simulink library "IOBlock_Library_TTC580"  (R2021a)
settings: Solver=ode45  StartTime=0.0  StopTime=10.0  RelTol=1e-3
PreLoadFcn:
  | addpath(genpath(fileparts(which('IOBlock_Library_TTC580'))));
  | %addpath(genpath(fileparts(which('IOBlock_Library_TTC580.mdl'))))
  | try
  | addpath(genpath([fileparts(which('IOBlock_Library_TTC580')),'\..\DBC_Importer']));
  | addpath(genpath([fileparts(which('IOBlock_Library_TTC580')),'\..\EEPROM_Importer']));
  | addpath(genpath([fileparts(which('IOBlock_Library_TTC580')),'\..\UserDoc']));
  | catch
  | warning('IOBlock_Library_TTC580: add path to DBC_Importer and EEPROM_Importer manually');
  | end
  | try
  | if exist('..\CustomPackage\scripts\OpenAllPackages.m','file')
  |      run('..\CustomPackage\scripts\OpenAllPackages.m'); %always available, ggf. empty
  | end
  | catch
  | warning('A problem occurred opening automatically the CustomPackage. Please open libraries manually');
  | end
  | try
  | set_param(0,'EditorSmartEditingHotParam','off');
  | catch
  | warning('Simlink preferences for ''Edit key parameter when adding new blocks'' needs to be unchecked manually');
  | end
undefined symbols (not defined in the file or in its folder): ADC_Absolute_10V, ADC_Absolute_32V, ADC_Absolute_5V, ADC_BoardTemp, ADC_ChannelInit, ADC_Current, ADC_Get, ADC_K15_, ADC_Ratiometric_10V, ADC_Ratiometric_5V, ADC_Resistive, ADC_SensorSupply, ADC_UBAT, bit_packing, bit_unpacking, CAN_ConfigMsg, compare2error, compare2FET_PROT_REENABLE, crc32_calc_intern, CRC32_EEPROM_Read, CRC32_EEPROM_Write, DIAG_EnterSafestate, DIAG_Status, DIAG_Status_internal, EEPROM_Mirror, EEPROM_Read, EEPROM_Read_OffsetIn, EEPROM_Read_Raw, EEPROM_Write, EEPROM_Write_OffsetIn, EEPROM_Write_Raw, EnterSafestate, FPU_Handler, Get_DI, Get_DI_VarThreshold, Get_K15_, Get_Pulse_Freq_Curr, Get_Pulse_Freq_Volt, Get_WakeUp, GetDateAndTime, IO_ADC_ResetProtection, IO_Blk_Lib_TTC500, IO_CAN_ReadMsg, IO_CAN_WriteMsg, IO_DI_Get, IO_DI_Init, IO_DI_Init_Var, IO_DO_GetCur, IO_DO_GetVoltage, IO_DO_Init, IO_DO_ResetProtection, IO_DO_Set, IO_Driver_GetSerialNumber, IO_Driver_GetVersionOfDriver, IO_Driver_GetVersionOfFPGA, IO_EEPROM_GetStatus, IO_EEPROM_Init, IO_EEPROM_Read_raw, IO_EEPROM_Write, IO_EEPROM_Write_OffsetIn ... (+73)
libraries: simulink x43
(part 10 of 18)

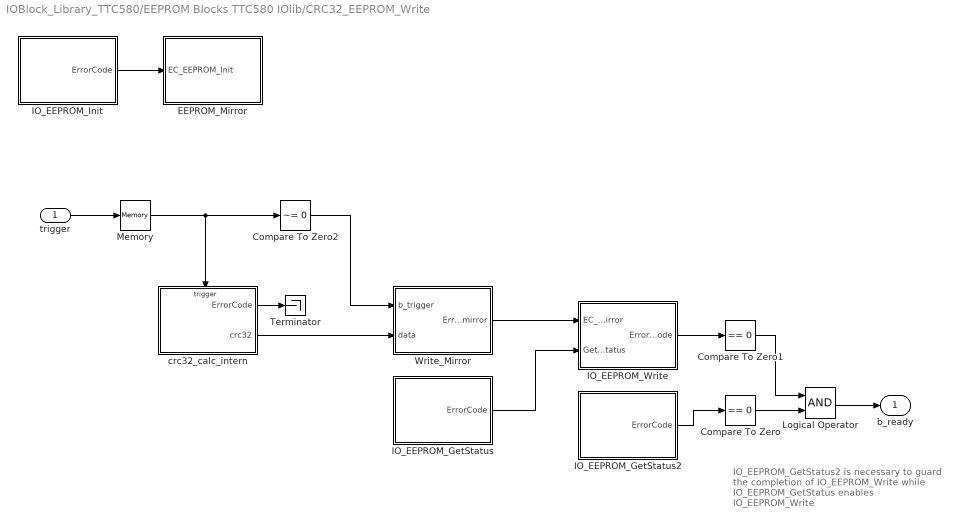
== system IOBlock_Library_TTC580/EEPROM Blocks TTC580 IOlib/CRC32_EEPROM_Write ==
  note: IO_EEPROM_GetStatus2 is necessary to
      | guard the completion of IO_EEPROM_Write
      | while IO_EEPROM_GetStatus enables
      | IO_EEPROM_Write
  trigger : Inport
  Compare To Zero : simulink/Logic and Bit Operations/Compare To Zero  relop===  OutDataTypeStr=boolean  ZeroCross=off
  Compare To Zero1 : simulink/Logic and Bit Operations/Compare To Zero  relop===  OutDataTypeStr=boolean  ZeroCross=off
  Compare To Zero2 : simulink/Logic and Bit Operations/Compare To Zero  relop=~=  OutDataTypeStr=boolean  ZeroCross=off
  EEPROM_Mirror : Subsystem  LoadFcn=|  mask(EEPROM_Mirror_Code){SampleTime=-1, ttlib=IO_Blk_Lib_TTC500, ttDescription=EEPROM_Mirror, tt_iolib_version=0.21, offset=0, length=65536}
      | try
      | %
      | %Upgrade Information - standard BEGIN
      | new_color = 'blue';
      | new_ver = '0.21';
      | act_ver = get_param(gcb,'tt_iolib_version');
      | if not(strcmp(act_ver,new_ver))
      |     disp(['Upgrade block: ',gcb,char(10),'       Version: ',act_ver,' -> ',new_ver]);
      |     %switch - case for specific upgrade information e.g. additional parameter required 
      |     %Change appearance and version information
      |     set_param(gcb,'ForegroundColor',new_color);
      |     set_param(gcb,'tt_iolib_version',new_ver);
      | end
      | %Upgrade Information - standard END
      | catch
      | %Standard catch section BEGIN 
      | disp(' ');
      | disp('------------------------------------------------------------');
      | disp('An error occurred in a callback of the TTC580-BlockLib.');
      | disp(['Please check the parameters in the mask of ',gcb]);
      | disp('If you do not encounter any violations, then please '); 
      | disp('copy the following lines and report this to support@ttcontrol.com ');
      | disp('<< begin of error message dump >>');
      | disp(['Version of TTC580-BlockLib: ', get_param(gcb,'tt_iolib_version')]);
      | disp(get_param(gcb,'ttDescription'));
      | disp(gcb);
      | x=lasterror;disp(x.message);
      | disp(get_param(gcb,'MaskValues'));
      | disp(version);
      | disp(computer);
      | disp('<< end of error message dump >>');
      | disp('------------------------------------------------------------');
      | disp(' ');
      | %Standard catch section END
      | end
      mask help:
      | Read all data from the EEPROM and mirror this onto RAM.
      | The ErrorCode of IO_EEPROM_Init - block must be connected to the input of EEPROM_Mirror.
      | After calling EEPROM_Mirror the global variable EEPROM_mirror is filled and
      | the global variable ErrorCode_EEPROM_mirror contains the returns of IO_EEPROM_Init() and IO_EEPROM_Read().
      mask init:
      | %
      settings: CopyFcn=%deleted
      mask Help: web(which('IO_EEPROM.h'))
      mask Callback offset: %
      mask Callback length: %
  IO_EEPROM_GetStatus : Subsystem  LoadFcn=|  mask(IO_EEPROM_GetStatus_Code){SampleTime=-1, ttlib=IO_Blk_Lib_TTC500, ttDescription=IO_EEPROM_GetStatus, tt_iolib_version=0.19}
      | try
      | %
      | %Upgrade Information - standard BEGIN
      | new_color = 'blue';
      | new_ver = '0.19';
      | act_ver = get_param(gcb,'tt_iolib_version');
      | if not(strcmp(act_ver,new_ver))
      |     disp(['Upgrade block: ',gcb,char(10),'       Version: ',act_ver,' -> ',new_ver]);
      |     %switch - case for specific upgrade information e.g. additional parameter required 
      |     %Change appearance and version information
      |     set_param(gcb,'ForegroundColor',new_color);
      |     set_param(gcb,'tt_iolib_version',new_ver);
      | end
      | %Upgrade Information - standard END
      | catch
      | %Standard catch section BEGIN 
      | disp(' ');
      | disp('------------------------------------------------------------');
      | disp('An error occurred in a callback of the TTC580-BlockLib.');
      | disp(['Please check the parameters in the mask of ',gcb]);
      | disp('If you do not encounter any violations, then please '); 
      | disp('copy the following lines and report this to support@ttcontrol.com ');
      | disp('<< begin of error message dump >>');
      | disp(['Version of TTC580-BlockLib: ', get_param(gcb,'tt_iolib_version')]);
      | disp(get_param(gcb,'ttDescription'));
      | disp(gcb);
      | x=lasterror;disp(x.message);
      | disp(get_param(gcb,'MaskValues'));
      | disp(version);
      | disp(computer);
      | disp('<< end of error message dump >>');
      | disp('------------------------------------------------------------');
      | disp(' ');
      | %Standard catch section END
      | end
      mask help: Returns the status of the EEPROM driver.
      mask init:
      | %
      settings: CopyFcn=%deleted
      mask Help: web(which('IO_EEPROM.h'))
  IO_EEPROM_GetStatus2 : Subsystem  LoadFcn=|  mask(IO_EEPROM_GetStatus_Code){SampleTime=-1, ttlib=IO_Blk_Lib_TTC500, ttDescription=IO_EEPROM_GetStatus, tt_iolib_version=0.19}
      | try
      | %
      | %Upgrade Information - standard BEGIN
      | new_color = 'blue';
      | new_ver = '0.19';
      | act_ver = get_param(gcb,'tt_iolib_version');
      | if not(strcmp(act_ver,new_ver))
      |     disp(['Upgrade block: ',gcb,char(10),'       Version: ',act_ver,' -> ',new_ver]);
      |     %switch - case for specific upgrade information e.g. additional parameter required 
      |     %Change appearance and version information
      |     set_param(gcb,'ForegroundColor',new_color);
      |     set_param(gcb,'tt_iolib_version',new_ver);
      | end
      | %Upgrade Information - standard END
      | catch
      | %Standard catch section BEGIN 
      | disp(' ');
      | disp('------------------------------------------------------------');
      | disp('An error occurred in a callback of the TTC580-BlockLib.');
      | disp('Please copy the following lines and report this to support@tttech.com ');
      | disp('<< begin of error message dump >>');
      | disp(['Version of TTC580-BlockLib: ', get_param(gcb,'tt_iolib_version')]);
      | disp(get_param(gcb,'ttDescription'));
      | disp(gcb);
      | x=lasterror;disp(x.message);
      | disp(get_param(gcb,'MaskValues'));
      | disp(version);
      | disp(computer);
      | disp('<< end of error message dump >>');
      | disp('------------------------------------------------------------');
      | disp(' ');
      | %Standard catch section END
      | end
      mask help: Returns the status of the EEPROM driver.
      mask init:
      | %
      settings: CopyFcn=%deleted
      mask Help: web(which('IO_EEPROM.h'))
  IO_EEPROM_Init : Subsystem  LoadFcn=|  mask(IO_EEPROM_Init_Code){SampleTime=-1, ttlib=IO_Blk_Lib_TTC500, ttDescription=IO_EEPROM_Init, tt_iolib_version=0.19}
      | try
      | %
      | %Upgrade Information - standard BEGIN
      | new_color = 'blue';
      | new_ver = '0.19';
      | act_ver = get_param(gcb,'tt_iolib_version');
      | if not(strcmp(act_ver,new_ver))
      |     disp(['Upgrade block: ',gcb,char(10),'       Version: ',act_ver,' -> ',new_ver]);
      |     %switch - case for specific upgrade information e.g. additional parameter required 
      |     %Change appearance and version information
      |     set_param(gcb,'ForegroundColor',new_color);
      |     set_param(gcb,'tt_iolib_version',new_ver);
      | end
      | %Upgrade Information - standard END
      | catch
      | %Standard catch section BEGIN 
      | disp(' ');
      | disp('------------------------------------------------------------');
      | disp('An error occurred in a callback of the TTC580-BlockLib.');
      | disp(['Please check the parameters in the mask of ',gcb]);
      | disp('If you do not encounter any violations, then please '); 
      | disp('copy the following lines and report this to support@ttcontrol.com ');
      | disp('<< begin of error message dump >>');
      | disp(['Version of TTC580-BlockLib: ', get_param(gcb,'tt_iolib_version')]);
      | disp(get_param(gcb,'ttDescription'));
      | disp(gcb);
      | x=lasterror;disp(x.message);
      | disp(get_param(gcb,'MaskValues'));
      | disp(version);
      | disp(computer);
      | disp('<< end of error message dump >>');
      | disp('------------------------------------------------------------');
      | disp(' ');
      | %Standard catch section END
      | end
      mask help: Initialization of the EEPROM driver.
      mask init:
      | %
      settings: CopyFcn=%deleted
      mask Help: web(which('IO_EEPROM.h'))
  IO_EEPROM_Write : Subsystem  LoadFcn=|  mask(IO_EEPROM_Write_Code){SampleTime=-1, ttlib=IO_Blk_Lib_TTC500, ttDescription=IO_EEPROM_Write, tt_iolib_version=0.19, offset=offset, length=length}
      | try
      | %
      | %Upgrade Information - standard BEGIN
      | new_color = 'blue';
      | new_ver = '0.19';
      | act_ver = get_param(gcb,'tt_iolib_version');
      | if not(strcmp(act_ver,new_ver))
      |     disp(['Upgrade block: ',gcb,char(10),'       Version: ',act_ver,' -> ',new_ver]);
      |     %switch - case for specific upgrade information e.g. additional parameter required 
      |     %Change appearance and version information
      |     set_param(gcb,'ForegroundColor',new_color);
      |     set_param(gcb,'tt_iolib_version',new_ver);
      | end
      | %Upgrade Information - standard END
      | catch
      | %Standard catch section BEGIN 
      | disp(' ');
      | disp('------------------------------------------------------------');
      | disp('An error occurred in a callback of the TTC580-BlockLib.');
      | disp(['Please check the parameters in the mask of ',gcb]);
      | disp('If you do not encounter any violations, then please '); 
      | disp('copy the following lines and report this to support@ttcontrol.com ');
      | disp('<< begin of error message dump >>');
      | disp(['Version of TTC580-BlockLib: ', get_param(gcb,'tt_iolib_version')]);
      | disp(get_param(gcb,'ttDescription'));
      | disp(gcb);
      | x=lasterror;disp(x.message);
      | disp(get_param(gcb,'MaskValues'));
      | disp(version);
      | disp(computer);
      | disp('<< end of error message dump >>');
      | disp('------------------------------------------------------------');
      | disp(' ');
      | %Standard catch section END
      | end
      mask help:
      | Copy data from EEPROM_mirror[] to physical EEPROM. Copy activity is triggered by the edge of the input "EC_Write_Mirror" from IO_E_BUSY to IO_E_OK.
      | The output "ErrorCode" is IO_E_BUSY as long as writing to EEPROM is pending. During the activities are performed writing to the physical EEPROM, "ErrorCode" corresponds to the output of the C-driver IO_EEPROM_Write().
      mask init:
      | %
      settings: CopyFcn=%deleted
      mask Help: web(which('IO_EEPROM.h'))
      mask Callback offset: %
      mask Callback length: %
  Logical Operator : Logic  AllPortsSameDT=off  OutDataTypeStr=boolean
  Memory : Memory  LinearizeAsDelay=on
  Terminator : Terminator
  Write_Mirror : Subsystem  LoadFcn=|  mask(Write_Mirror_Code){SampleTime=-1, ttlib=IO_Blk_Lib_TTC500, ttDescription=Write_Mirror, tt_iolib_version=0.19, offset=offset, length=length}
      | try
      | %
      | %Upgrade Information - standard BEGIN
      | new_color = 'blue';
      | new_ver = '0.19';
      | act_ver = get_param(gcb,'tt_iolib_version');
      | if not(strcmp(act_ver,new_ver))
      |     disp(['Upgrade block: ',gcb,char(10),'       Version: ',act_ver,' -> ',new_ver]);
      |     %switch - case for specific upgrade information e.g. additional parameter required 
      |     %Change appearance and version information
      |     set_param(gcb,'ForegroundColor',new_color);
      |     set_param(gcb,'tt_iolib_version',new_ver);
      | end
      | %Upgrade Information - standard END
      | catch
      | %Standard catch section BEGIN 
      | disp(' ');
      | disp('------------------------------------------------------------');
      | disp('An error occurred in a callback of the TTC580-BlockLib.');
      | disp(['Please check the parameters in the mask of ',gcb]);
      | disp('If you do not encounter any violations, then please '); 
      | disp('copy the following lines and report this to support@ttcontrol.com ');
      | disp('<< begin of error message dump >>');
      | disp(['Version of TTC580-BlockLib: ', get_param(gcb,'tt_iolib_version')]);
      | disp(get_param(gcb,'ttDescription'));
      | disp(gcb);
      | x=lasterror;disp(x.message);
      | disp(get_param(gcb,'MaskValues'));
      | disp(version);
      | disp(computer);
      | disp('<< end of error message dump >>');
      | disp('------------------------------------------------------------');
      | disp(' ');
      | %Standard catch section END
      | end
      mask help:
      | Write data to the mirror of the EEPROM. ErrorCode is set to IO_E_BUSY for one cycle of writing into EEPROM_mirror[].
      | In case the given data section exceeds given EEPROM boundaries, IO_E_EEPROM_RANGE ErrorCode is returned.
      mask init:
      | %
      settings: CopyFcn=%deleted
      mask Help: web(which('~.h'))
      mask Callback offset: %
      mask Callback length: %
  crc32_calc_intern : Subsystem  LoadFcn=|  mask(crc32_calc_intern_Code){SampleTime=-1, ttlib=IO_Blk_Lib_TTC500, ttDescription=crc32_calc_intern, tt_iolib_version=0.19, EEPROM_mirror=EEPROM_mirror, iBasicAddr_intern=BasicAddr, iEndAddr_intern=EndAddr}
      | try
      | %
      | %Upgrade Information - standard BEGIN
      | new_color = 'blue';
      | new_ver = '0.19';
      | act_ver = get_param(gcb,'tt_iolib_version');
      | if not(strcmp(act_ver,new_ver))
      |     disp(['Upgrade block: ',gcb,char(10),'       Version: ',act_ver,' -> ',new_ver]);
      |     %switch - case for specific upgrade information e.g. additional parameter required 
      |     %Change appearance and version information
      |     set_param(gcb,'ForegroundColor',new_color);
      |     set_param(gcb,'tt_iolib_version',new_ver);
      | end
      | %Upgrade Information - standard END
      | catch
      | %Standard catch section BEGIN 
      | disp(' ');
      | disp('------------------------------------------------------------');
      | disp('An error occurred in a callback of the TTC580-BlockLib.');
      | disp(['Please check the parameters in the mask of ',gcb]);
      | disp('If you do not encounter any violations, then please '); 
      | disp('copy the following lines and report this to support@ttcontrol.com ');
      | disp('<< begin of error message dump >>');
      | disp(['Version of TTC580-BlockLib: ', get_param(gcb,'tt_iolib_version')]);
      | disp(get_param(gcb,'ttDescription'));
      | disp(gcb);
      | x=lasterror;disp(x.message);
      | disp(get_param(gcb,'MaskValues'));
      | disp(version);
      | disp(computer);
      | disp('<< end of error message dump >>');
      | disp('------------------------------------------------------------');
      | disp(' ');
      | %Standard catch section END
      | end
      mask help:
      | Calculate crc32 for a section out of the EEPROM.
      | In case the given data section exceeds given EEPROM boundaries, non zero ErrorCode is returned.
      mask init:
      | %
      settings: CopyFcn=%deleted
      mask Help: No further help available for this block
      mask Callback EEPROM_mirror: %
      mask Callback iBasicAddr_intern: %
      mask Callback iEndAddr_intern: %
  b_ready : Outport  VectorParamsAs1DForOutWhenUnconnected=off
  wires:
  IO_EEPROM_GetStatus2/1(ErrorCode) -> Compare To Zero/1
  Compare To Zero/1 -> Logical Operator/2
  crc32_calc_intern/1(ErrorCode) -> Terminator/1
  Logical Operator/1 -> b_ready/1
  Compare To Zero1/1 -> Logical Operator/1
  Memory/1 -> crc32_calc_intern/Trigger, Compare To Zero2/1
  Compare To Zero2/1 -> Write_Mirror/1(b_trigger)
  crc32_calc_intern/2(crc32) -> Write_Mirror/2(data)
  IO_EEPROM_GetStatus/1(ErrorCode) -> IO_EEPROM_Write/2(GetStatus)
  Write_Mirror/1(ErrorCode_EEPROM_mirror) -> IO_EEPROM_Write/1(EC_Write_Mirror)
  trigger/1 -> Memory/1
  IO_EEPROM_Write/1(ErrorCode) -> Compare To Zero1/1
  IO_EEPROM_Init/1(ErrorCode) -> EEPROM_Mirror/1(EC_EEPROM_Init)

== system IOBlock_Library_TTC580/EEPROM Blocks TTC580 IOlib/EEPROM_Read ==
  Compare To Zero1 : simulink/Logic and Bit Operations/Compare To Zero  relop===  OutDataTypeStr=boolean  ZeroCross=off
  Compare To Zero2 : simulink/Logic and Bit Operations/Compare To Zero  relop===  OutDataTypeStr=boolean  ZeroCross=off
  EEPROM_Mirror : Subsystem  LoadFcn=|  mask(EEPROM_Mirror_Code){SampleTime=-1, ttlib=IO_Blk_Lib_TTC500, ttDescription=EEPROM_Mirror, tt_iolib_version=0.21, offset=0, length=65536}
      | try
      | %
      | %Upgrade Information - standard BEGIN
      | new_color = 'blue';
      | new_ver = '0.21';
      | act_ver = get_param(gcb,'tt_iolib_version');
      | if not(strcmp(act_ver,new_ver))
      |     disp(['Upgrade block: ',gcb,char(10),'       Version: ',act_ver,' -> ',new_ver]);
      |     %switch - case for specific upgrade information e.g. additional parameter required 
      |     %Change appearance and version information
      |     set_param(gcb,'ForegroundColor',new_color);
      |     set_param(gcb,'tt_iolib_version',new_ver);
      | end
      | %Upgrade Information - standard END
      | catch
      | %Standard catch section BEGIN 
      | disp(' ');
      | disp('------------------------------------------------------------');
      | disp('An error occurred in a callback of the TTC580-BlockLib.');
      | disp(['Please check the parameters in the mask of ',gcb]);
      | disp('If you do not encounter any violations, then please '); 
      | disp('copy the following lines and report this to support@ttcontrol.com ');
      | disp('<< begin of error message dump >>');
      | disp(['Version of TTC580-BlockLib: ', get_param(gcb,'tt_iolib_version')]);
      | disp(get_param(gcb,'ttDescription'));
      | disp(gcb);
      | x=lasterror;disp(x.message);
      | disp(get_param(gcb,'MaskValues'));
      | disp(version);
      | disp(computer);
      | disp('<< end of error message dump >>');
      | disp('------------------------------------------------------------');
      | disp(' ');
      | %Standard catch section END
      | end
      mask help:
      | Read all data from the EEPROM and mirror this onto RAM.
      | The ErrorCode of IO_EEPROM_Init - block must be connected to the input of EEPROM_Mirror.
      | After calling EEPROM_Mirror the global variable EEPROM_mirror is filled and
      | the global variable ErrorCode_EEPROM_mirror contains the returns of IO_EEPROM_Init() and IO_EEPROM_Read().
      mask init:
      | %
      settings: CopyFcn=%deleted
      mask Help: web(which('IO_EEPROM.h'))
      mask Callback offset: %
      mask Callback length: %
  IO_EEPROM_GetStatus : Subsystem  LoadFcn=|  mask(IO_EEPROM_GetStatus_Code){SampleTime=-1, ttlib=IO_Blk_Lib_TTC500, ttDescription=IO_EEPROM_GetStatus, tt_iolib_version=0.19}
      | try
      | %
      | %Upgrade Information - standard BEGIN
      | new_color = 'blue';
      | new_ver = '0.19';
      | act_ver = get_param(gcb,'tt_iolib_version');
      | if not(strcmp(act_ver,new_ver))
      |     disp(['Upgrade block: ',gcb,char(10),'       Version: ',act_ver,' -> ',new_ver]);
      |     %switch - case for specific upgrade information e.g. additional parameter required 
      |     %Change appearance and version information
      |     set_param(gcb,'ForegroundColor',new_color);
      |     set_param(gcb,'tt_iolib_version',new_ver);
      | end
      | %Upgrade Information - standard END
      | catch
      | %Standard catch section BEGIN 
      | disp(' ');
      | disp('------------------------------------------------------------');
      | disp('An error occurred in a callback of the TTC580-BlockLib.');
      | disp(['Please check the parameters in the mask of ',gcb]);
      | disp('If you do not encounter any violations, then please '); 
      | disp('copy the following lines and report this to support@ttcontrol.com ');
      | disp('<< begin of error message dump >>');
      | disp(['Version of TTC580-BlockLib: ', get_param(gcb,'tt_iolib_version')]);
      | disp(get_param(gcb,'ttDescription'));
      | disp(gcb);
      | x=lasterror;disp(x.message);
      | disp(get_param(gcb,'MaskValues'));
      | disp(version);
      | disp(computer);
      | disp('<< end of error message dump >>');
      | disp('------------------------------------------------------------');
      | disp(' ');
      | %Standard catch section END
      | end
      mask help: Returns the status of the EEPROM driver.
      mask init:
      | %
      settings: CopyFcn=%deleted
      mask Help: web(which('IO_EEPROM.h'))
  IO_EEPROM_Init : Subsystem  LoadFcn=|  mask(IO_EEPROM_Init_Code){SampleTime=-1, ttlib=IO_Blk_Lib_TTC500, ttDescription=IO_EEPROM_Init, tt_iolib_version=0.19}
      | try
      | %
      | %Upgrade Information - standard BEGIN
      | new_color = 'blue';
      | new_ver = '0.19';
      | act_ver = get_param(gcb,'tt_iolib_version');
      | if not(strcmp(act_ver,new_ver))
      |     disp(['Upgrade block: ',gcb,char(10),'       Version: ',act_ver,' -> ',new_ver]);
      |     %switch - case for specific upgrade information e.g. additional parameter required 
      |     %Change appearance and version information
      |     set_param(gcb,'ForegroundColor',new_color);
      |     set_param(gcb,'tt_iolib_version',new_ver);
      | end
      | %Upgrade Information - standard END
      | catch
      | %Standard catch section BEGIN 
      | disp(' ');
      | disp('------------------------------------------------------------');
      | disp('An error occurred in a callback of the TTC580-BlockLib.');
      | disp(['Please check the parameters in the mask of ',gcb]);
      | disp('If you do not encounter any violations, then please '); 
      | disp('copy the following lines and report this to support@ttcontrol.com ');
      | disp('<< begin of error message dump >>');
      | disp(['Version of TTC580-BlockLib: ', get_param(gcb,'tt_iolib_version')]);
      | disp(get_param(gcb,'ttDescription'));
      | disp(gcb);
      | x=lasterror;disp(x.message);
      | disp(get_param(gcb,'MaskValues'));
      | disp(version);
      | disp(computer);
      | disp('<< end of error message dump >>');
      | disp('------------------------------------------------------------');
      | disp(' ');
      | %Standard catch section END
      | end
      mask help: Initialization of the EEPROM driver.
      mask init:
      | %
      settings: CopyFcn=%deleted
      mask Help: web(which('IO_EEPROM.h'))
  Logical Operator : Logic  AllPortsSameDT=off  OutDataTypeStr=boolean
  Read_Mirror : Subsystem  LoadFcn=|  mask(Read_Mirror_Code){SampleTime=-1, ttlib=IO_Blk_Lib_TTC500, ttDescription=Read_Mirror, tt_iolib_version=0.19, offset=offset, length=length}
      | try
      | %
      | %Upgrade Information - standard BEGIN
      | new_color = 'blue';
      | new_ver = '0.19';
      | act_ver = get_param(gcb,'tt_iolib_version');
      | if not(strcmp(act_ver,new_ver))
      |     disp(['Upgrade block: ',gcb,char(10),'       Version: ',act_ver,' -> ',new_ver]);
      |     %switch - case for specific upgrade information e.g. additional parameter required 
      |     %Change appearance and version information
      |     set_param(gcb,'ForegroundColor',new_color);
      |     set_param(gcb,'tt_iolib_version',new_ver);
      | end
      | %Upgrade Information - standard END
      | catch
      | %Standard catch section BEGIN 
      | disp(' ');
      | disp('------------------------------------------------------------');
      | disp('An error occurred in a callback of the TTC580-BlockLib.');
      | disp(['Please check the parameters in the mask of ',gcb]);
      | disp('If you do not encounter any violations, then please '); 
      | disp('copy the following lines and report this to support@ttcontrol.com ');
      | disp('<< begin of error message dump >>');
      | disp(['Version of TTC580-BlockLib: ', get_param(gcb,'tt_iolib_version')]);
      | disp(get_param(gcb,'ttDescription'));
      | disp(gcb);
      | x=lasterror;disp(x.message);
      | disp(get_param(gcb,'MaskValues'));
      | disp(version);
      | disp(computer);
      | disp('<< end of error message dump >>');
      | disp('------------------------------------------------------------');
      | disp(' ');
      | %Standard catch section END
      | end
      mask help:
      | Read data from the mirror of the EEPROM.
      | In case the given data section exceeds given EEPROM boundaries, IO_E_EEPROM_RANGE ErrorCode is returned.
      mask init:
      | %
      settings: CopyFcn=%deleted
      mask Help: web(which('~.h'))
      mask Callback offset: %
      mask Callback length: %
  once_true: Mirror filled : Subsystem  mask(SRFlipFlop){initial_condition=0}
      mask prompts: initial_condition "Initial condition (state of Q):"
      mask help: S-R Flip-Flop Block
      mask Help:
      | The S-R flip-flop also known as a set-reset flip-flop. This implementation
      | is modeled after an S-R flip-flop constructed using NOR gates. The
      | truth table for this block is:
      | <pre>
      |  S  R   Q  !Q
      |  ----------------
      |  1  0   1  0
      |  0  0   1  0  (after S == 1, R == 0)
      |  0  1   0  1
      |  0  0   0  1  (after S == 0, R == 1)
      |  1  1   0  0
      | </pre>
      | 
      | In an S-R flip-flop that is implemented with NOR gates, when a 1 is
      | applied to both the set and reset inputs, both outputs go to 0. Technically,
      | this state is undefined and is usually avoided. Note, if the flip-flop is
      | implemented with NAND gates, when a 0 is applied to both inputs, both outputs
      | go to 0 and when a 1 is applied to both inputs, the output depends on
      | the previous state of the flip-flop (previous value of Q).
  b_ready : Outport  VectorParamsAs1DForOutWhenUnconnected=off
  data : Outport  Port=2  OutDataTypeStr=EEPROM_type  VectorParamsAs1DForOutWhenUnconnected=off
  wires:
  Read_Mirror/2(data) -> data/1
  Read_Mirror/1(ErrorCode_EEPROM_mirror) -> Compare To Zero1/1
  IO_EEPROM_Init/1(ErrorCode) -> EEPROM_Mirror/1(EC_EEPROM_Init)
  IO_EEPROM_GetStatus/1(ErrorCode) -> Compare To Zero2/1
  Logical Operator/1 -> b_ready/1
  Compare To Zero1/1 -> Logical Operator/2
  Compare To Zero2/1 -> once_true: Mirror filled/1(S)
  once_true: Mirror filled/1(Q) -> Logical Operator/1

== system IOBlock_Library_TTC580/EEPROM Blocks TTC580 IOlib/EEPROM_Read_OffsetIn ==
  offset : Inport  OutDataTypeStr=uint16  PortDimensions=1
  Compare To Zero1 : simulink/Logic and Bit Operations/Compare To Zero  relop===  OutDataTypeStr=boolean  ZeroCross=off
  Compare To Zero2 : simulink/Logic and Bit Operations/Compare To Zero  relop===  OutDataTypeStr=boolean  ZeroCross=off
  EEPROM_Mirror : Subsystem  LoadFcn=|  mask(EEPROM_Mirror_Code){SampleTime=-1, ttlib=IO_Blk_Lib_TTC500, ttDescription=EEPROM_Mirror, tt_iolib_version=0.21, offset=0, length=65536}
      | try
      | %
      | %Upgrade Information - standard BEGIN
      | new_color = 'blue';
      | new_ver = '0.21';
      | act_ver = get_param(gcb,'tt_iolib_version');
      | if not(strcmp(act_ver,new_ver))
      |     disp(['Upgrade block: ',gcb,char(10),'       Version: ',act_ver,' -> ',new_ver]);
      |     %switch - case for specific upgrade information e.g. additional parameter required 
      |     %Change appearance and version information
      |     set_param(gcb,'ForegroundColor',new_color);
      |     set_param(gcb,'tt_iolib_version',new_ver);
      | end
      | %Upgrade Information - standard END
      | catch
      | %Standard catch section BEGIN 
      | disp(' ');
      | disp('------------------------------------------------------------');
      | disp('An error occurred in a callback of the TTC580-BlockLib.');
      | disp(['Please check the parameters in the mask of ',gcb]);
      | disp('If you do not encounter any violations, then please '); 
      | disp('copy the following lines and report this to support@ttcontrol.com ');
      | disp('<< begin of error message dump >>');
      | disp(['Version of TTC580-BlockLib: ', get_param(gcb,'tt_iolib_version')]);
      | disp(get_param(gcb,'ttDescription'));
      | disp(gcb);
      | x=lasterror;disp(x.message);
      | disp(get_param(gcb,'MaskValues'));
      | disp(version);
      | disp(computer);
      | disp('<< end of error message dump >>');
      | disp('------------------------------------------------------------');
      | disp(' ');
      | %Standard catch section END
      | end
      mask help:
      | Read all data from the EEPROM and mirror this onto RAM.
      | The ErrorCode of IO_EEPROM_Init - block must be connected to the input of EEPROM_Mirror.
      | After calling EEPROM_Mirror the global variable EEPROM_mirror is filled and
      | the global variable ErrorCode_EEPROM_mirror contains the returns of IO_EEPROM_Init() and IO_EEPROM_Read().
      mask init:
      | %
      settings: CopyFcn=%deleted
      mask Help: web(which('IO_EEPROM.h'))
      mask Callback offset: %
      mask Callback length: %
  IO_EEPROM_GetStatus : Subsystem  LoadFcn=|  mask(IO_EEPROM_GetStatus_Code){SampleTime=-1, ttlib=IO_Blk_Lib_TTC500, ttDescription=IO_EEPROM_GetStatus, tt_iolib_version=0.19}
      | try
      | %
      | %Upgrade Information - standard BEGIN
      | new_color = 'blue';
      | new_ver = '0.19';
      | act_ver = get_param(gcb,'tt_iolib_version');
      | if not(strcmp(act_ver,new_ver))
      |     disp(['Upgrade block: ',gcb,char(10),'       Version: ',act_ver,' -> ',new_ver]);
      |     %switch - case for specific upgrade information e.g. additional parameter required 
      |     %Change appearance and version information
      |     set_param(gcb,'ForegroundColor',new_color);
      |     set_param(gcb,'tt_iolib_version',new_ver);
      | end
      | %Upgrade Information - standard END
      | catch
      | %Standard catch section BEGIN 
      | disp(' ');
      | disp('------------------------------------------------------------');
      | disp('An error occurred in a callback of the TTC580-BlockLib.');
      | disp(['Please check the parameters in the mask of ',gcb]);
      | disp('If you do not encounter any violations, then please '); 
      | disp('copy the following lines and report this to support@ttcontrol.com ');
      | disp('<< begin of error message dump >>');
      | disp(['Version of TTC580-BlockLib: ', get_param(gcb,'tt_iolib_version')]);
      | disp(get_param(gcb,'ttDescription'));
      | disp(gcb);
      | x=lasterror;disp(x.message);
      | disp(get_param(gcb,'MaskValues'));
      | disp(version);
      | disp(computer);
      | disp('<< end of error message dump >>');
      | disp('------------------------------------------------------------');
      | disp(' ');
      | %Standard catch section END
      | end
      mask help: Returns the status of the EEPROM driver.
      mask init:
      | %
      settings: CopyFcn=%deleted
      mask Help: web(which('IO_EEPROM.h'))
  IO_EEPROM_Init : Subsystem  LoadFcn=|  mask(IO_EEPROM_Init_Code){SampleTime=-1, ttlib=IO_Blk_Lib_TTC500, ttDescription=IO_EEPROM_Init, tt_iolib_version=0.19}
      | try
      | %
      | %Upgrade Information - standard BEGIN
      | new_color = 'blue';
      | new_ver = '0.19';
      | act_ver = get_param(gcb,'tt_iolib_version');
      | if not(strcmp(act_ver,new_ver))
      |     disp(['Upgrade block: ',gcb,char(10),'       Version: ',act_ver,' -> ',new_ver]);
      |     %switch - case for specific upgrade information e.g. additional parameter required 
      |     %Change appearance and version information
      |     set_param(gcb,'ForegroundColor',new_color);
      |     set_param(gcb,'tt_iolib_version',new_ver);
      | end
      | %Upgrade Information - standard END
      | catch
      | %Standard catch section BEGIN 
      | disp(' ');
      | disp('------------------------------------------------------------');
      | disp('An error occurred in a callback of the TTC580-BlockLib.');
      | disp(['Please check the parameters in the mask of ',gcb]);
      | disp('If you do not encounter any violations, then please '); 
      | disp('copy the following lines and report this to support@ttcontrol.com ');
      | disp('<< begin of error message dump >>');
      | disp(['Version of TTC580-BlockLib: ', get_param(gcb,'tt_iolib_version')]);
      | disp(get_param(gcb,'ttDescription'));
      | disp(gcb);
      | x=lasterror;disp(x.message);
      | disp(get_param(gcb,'MaskValues'));
      | disp(version);
      | disp(computer);
      | disp('<< end of error message dump >>');
      | disp('------------------------------------------------------------');
      | disp(' ');
      | %Standard catch section END
      | end
      mask help: Initialization of the EEPROM driver.
      mask init:
      | %
      settings: CopyFcn=%deleted
      mask Help: web(which('IO_EEPROM.h'))
  Logical Operator : Logic  AllPortsSameDT=off  OutDataTypeStr=boolean
  Read_Mirror_OffsetIn : Subsystem  LoadFcn=|  mask(Read_Mirror_OffsetIn_Code){SampleTime=-1, ttlib=IO_Blk_Lib_TTC500, ttDescription=Read_Mirror_OffsetIn, tt_iolib_version=0.23, length=length}
      | try
      | %
      | %Upgrade Information - standard BEGIN
      | new_color = 'blue';
      | new_ver = '0.23';
      | act_ver = get_param(gcb,'tt_iolib_version');
      | if not(strcmp(act_ver,new_ver))
      |     disp(['Upgrade block: ',gcb,char(10),'       Version: ',act_ver,' -> ',new_ver]);
      |     %switch - case for specific upgrade information e.g. additional parameter required 
      |     %Change appearance and version information
      |     set_param(gcb,'ForegroundColor',new_color);
      |     set_param(gcb,'tt_iolib_version',new_ver);
      | end
      | %Upgrade Information - standard END
      | catch
      | %Standard catch section BEGIN 
      | disp(' ');
      | disp('------------------------------------------------------------');
      | disp('An error occurred in a callback of the TTC580-BlockLib.');
      | disp(['Please check the parameters in the mask of ',gcb]);
      | disp('If you do not encounter any violations, then please '); 
      | disp('copy the following lines and report this to support@ttcontrol.com ');
      | disp('<< begin of error message dump >>');
      | disp(['Version of TTC580-BlockLib: ', get_param(gcb,'tt_iolib_version')]);
      | disp(get_param(gcb,'ttDescription'));
      | disp(gcb);
      | x=lasterror;disp(x.message);
      | disp(get_param(gcb,'MaskValues'));
      | disp(version);
      | disp(computer);
      | disp('<< end of error message dump >>');
      | disp('------------------------------------------------------------');
      | disp(' ');
      | %Standard catch section END
      | end
      mask help:
      | Read data from the mirror of the EEPROM.
      | In case the given data section exceeds given EEPROM boundaries, IO_E_EEPROM_RANGE ErrorCode is returned.
      mask init:
      | %
      settings: CopyFcn=%deleted
      mask Help: No further help available for this block
      mask Callback length: %
  once_true: Mirror filled : Subsystem  mask(SRFlipFlop){initial_condition=0}
      mask prompts: initial_condition "Initial condition (state of Q):"
      mask help: S-R Flip-Flop Block
      mask Help:
      | The S-R flip-flop also known as a set-reset flip-flop. This implementation
      | is modeled after an S-R flip-flop constructed using NOR gates. The
      | truth table for this block is:
      | <pre>
      |  S  R   Q  !Q
      |  ----------------
      |  1  0   1  0
      |  0  0   1  0  (after S == 1, R == 0)
      |  0  1   0  1
      |  0  0   0  1  (after S == 0, R == 1)
      |  1  1   0  0
      | </pre>
      | 
      | In an S-R flip-flop that is implemented with NOR gates, when a 1 is
      | applied to both the set and reset inputs, both outputs go to 0. Technically,
      | this state is undefined and is usually avoided. Note, if the flip-flop is
      | implemented with NAND gates, when a 0 is applied to both inputs, both outputs
      | go to 0 and when a 1 is applied to both inputs, the output depends on
      | the previous state of the flip-flop (previous value of Q).
  b_ready : Outport  VectorParamsAs1DForOutWhenUnconnected=off
  data : Outport  Port=2  OutDataTypeStr=EEPROM_type  VectorParamsAs1DForOutWhenUnconnected=off
  wires:
  Read_Mirror_OffsetIn/2(data) -> data/1
  Read_Mirror_OffsetIn/1(ErrorCode_EEPROM_mirror) -> Compare To Zero1/1
  IO_EEPROM_Init/1(ErrorCode) -> EEPROM_Mirror/1(EC_EEPROM_Init)
  IO_EEPROM_GetStatus/1(ErrorCode) -> Compare To Zero2/1
  Logical Operator/1 -> b_ready/1
  Compare To Zero2/1 -> once_true: Mirror filled/1(S)
  Compare To Zero1/1 -> Logical Operator/2
  offset/1 -> Read_Mirror_OffsetIn/1(offset)
  once_true: Mirror filled/1(Q) -> Logical Operator/1

== system IOBlock_Library_TTC580/EEPROM Blocks TTC580 IOlib/EEPROM_Read_Raw ==
  IO_EEPROM_Init : Subsystem  LoadFcn=|  mask(IO_EEPROM_Init_Code){SampleTime=-1, ttlib=IO_Blk_Lib_TTC500, ttDescription=IO_EEPROM_Init, tt_iolib_version=0.24}
      | try
      | %
      | %Upgrade Information - standard BEGIN
      | new_color = 'blue';
      | new_ver = '0.24';
      | act_ver = get_param(gcb,'tt_iolib_version');
      | if not(strcmp(act_ver,new_ver))
      |     disp(['Upgrade block: ',gcb,char(10),'       Version: ',act_ver,' -> ',new_ver]);
      |     %switch - case for specific upgrade information e.g. additional parameter required 
      |     %Change appearance and version information
      |     set_param(gcb,'ForegroundColor',new_color);
      |     set_param(gcb,'tt_iolib_version',new_ver);
      | end
      | %Upgrade Information - standard END
      | catch
      | %Standard catch section BEGIN 
      | disp(' ');
      | disp('------------------------------------------------------------');
      | disp('An error occurred in a callback of the TTC580-BlockLib.');
      | disp(['Please check the parameters in the mask of ',gcb]);
      | disp('If you do not encounter any violations, then please '); 
      | disp('copy the following lines and report this to support@ttcontrol.com ');
      | disp('<< begin of error message dump >>');
      | disp(['Version of TTC580-BlockLib: ', get_param(gcb,'tt_iolib_version')]);
      | disp(get_param(gcb,'ttDescription'));
      | disp(gcb);
      | x=lasterror;disp(x.message);
      | disp(get_param(gcb,'MaskValues'));
      | disp(version);
      | disp(computer);
      | disp('<< end of error message dump >>');
      | disp('------------------------------------------------------------');
      | disp(' ');
      | %Standard catch section END
      | end
      mask help: Initialization of the EEPROM driver.
      mask init:
      | %
      settings: CopyFcn=%deleted
      mask Help: No further help available for this block
  IO_EEPROM_Read_raw : Subsystem  LoadFcn=|  mask(IO_EEPROM_Read_raw_Code){SampleTime=-1, ttlib=IO_Blk_Lib_TTC500, ttDescription=IO_EEPROM_Read_raw, tt_iolib_version=0.24, offset=offset, length=length}
      | try
      | %
      | %Upgrade Information - standard BEGIN
      | new_color = 'blue';
      | new_ver = '0.24';
      | act_ver = get_param(gcb,'tt_iolib_version');
      | if not(strcmp(act_ver,new_ver))
      |     disp(['Upgrade block: ',gcb,char(10),'       Version: ',act_ver,' -> ',new_ver]);
      |     %switch - case for specific upgrade information e.g. additional parameter required 
      |     %Change appearance and version information
      |     set_param(gcb,'ForegroundColor',new_color);
      |     set_param(gcb,'tt_iolib_version',new_ver);
      | end
      | %Upgrade Information - standard END
      | catch
      | %Standard catch section BEGIN 
      | disp(' ');
      | disp('------------------------------------------------------------');
      | disp('An error occurred in a callback of the TTC580-BlockLib.');
      | disp(['Please check the parameters in the mask of ',gcb]);
      | disp('If you do not encounter any violations, then please '); 
      | disp('copy the following lines and report this to support@ttcontrol.com ');
      | disp('<< begin of error message dump >>');
      | disp(['Version of TTC580-BlockLib: ', get_param(gcb,'tt_iolib_version')]);
      | disp(get_param(gcb,'ttDescription'));
      | disp(gcb);
      | x=lasterror;disp(x.message);
      | disp(get_param(gcb,'MaskValues'));
      | disp(version);
      | disp(computer);
      | disp('<< end of error message dump >>');
      | disp('------------------------------------------------------------');
      | disp(' ');
      | %Standard catch section END
      | end
      mask help: Read data from the EEPROM.
      mask init:
      | %
      settings: CopyFcn=%deleted
      mask Help: No further help available for this block
      mask Callback offset: %
      mask Callback length: %
  Terminator : Terminator
  ErrorCode : Outport  VectorParamsAs1DForOutWhenUnconnected=off
  data : Outport  Port=2  OutDataTypeStr=EEPROM_type  VectorParamsAs1DForOutWhenUnconnected=off
  wires:
  IO_EEPROM_Init/1(ErrorCode) -> Terminator/1
  IO_EEPROM_Read_raw/2(data) -> data/1
  IO_EEPROM_Read_raw/1(ErrorCode) -> ErrorCode/1
